simulink model "SigProc"  (R2020b)
settings: Solver=FixedStepDiscrete  StartTime=0.0  StopTime=10  RelTol=1e-3
values from neighbouring files (symbols this model uses):
  dt = 1/Fs    (= 0.1)    [OverSmp.m]    (also in dsp_assist.m = 1e-06; signal_analysis.m = 0.001)
libraries: commdigbbndpm3 x1, commrandsrc3 x1, dspsrcs4 x1
settings Model: Creator=User  LastModifiedBy=User

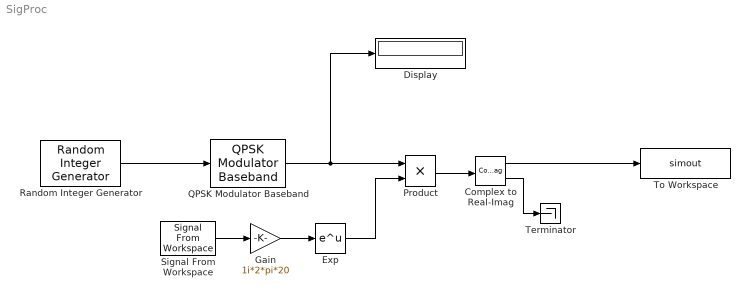
== system SigProc ==
  Complex to Real-Imag : ComplexToRealImag
  Display : Display
  Exp : Math  SaturateOnIntegerOverflow=on
  Gain : Gain  Gain=1i*2*pi*20
  Product : Product
  QPSK Modulator Baseband : commdigbbndpm3/QPSK Modulator Baseband  InType=Integer  Enc=Gray  Ph=pi/4  outDtype=double  outWordLen=16  outUDDataType=sfix(16)  outFracLenMode=Best precision  outFracLen=15  outDataTypeStr=double  outLastDataTypeStr=double
      settings: SourceProductName=Communications Toolbox
  Random Integer Generator : commrandsrc3/Random Integer Generator  SetSize=4  SeedSource=Auto  Seed=0  SampleTime=dt  SamplesPerFrame=1  OutputDataType=double  SimulateUsing=Interpreted execution
  Signal From Workspace : dspsrcs4/Signal From Workspace  X=t  Ts=dt  nsamps=1  OutputAfterFinalValue=Cyclic repetition  ignoreOrWarnInputAndFrameLengths=off  OutputFrames=off
  Terminator : Terminator
  To Workspace : ToWorkspace  VariableName=simout  SampleTime=dt
      settings: Save2DSignal=2-D array (concatenate along first dimension)
  wires:
  Random Integer Generator/1 -> QPSK Modulator Baseband/1
  QPSK Modulator Baseband/1 -> Product/1, Display/1
  Signal From Workspace/1 -> Gain/1
  Gain/1 -> Exp/1
  Exp/1 -> Product/2
  Product/1 -> Complex to Real-Imag/1
  Complex to Real-Imag/2 -> Terminator/1
  Complex to Real-Imag/1 -> To Workspace/1
